simulink subsystem "Global_2_Local_Path"  (R2022b)
settings: Solver=VariableStepAuto  StartTime=0.0  StopTime=10.0  RelTol=1e-3
settings Model: Creator=User  LastModifiedBy=User

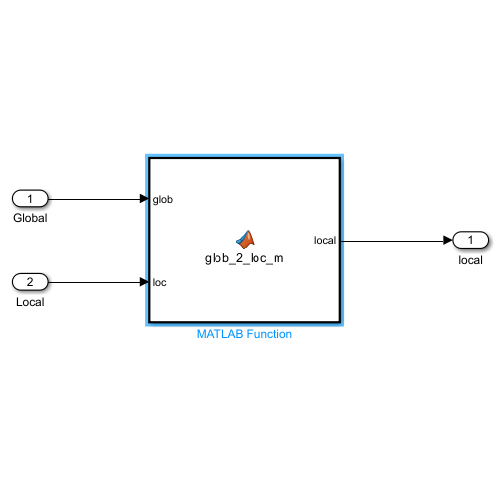
[thumbnail: Simulink's stored preview of the top-level diagram]
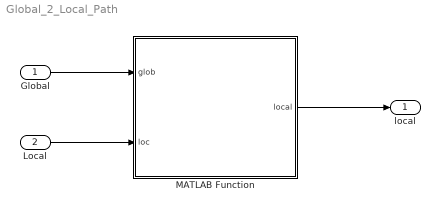
== system Global_2_Local_Path ==
  Global : Inport
  Local : Inport  Port=2
  MATLAB Function : MATLAB Function  TreatAsAtomicUnit=on
  local : Outport
  wires:
  Global/1 -> MATLAB Function/1(glob)
  Local/1 -> MATLAB Function/2(loc)
  MATLAB Function/1(local) -> local/1

== matlab function Global_2_Local_Path/MATLAB Function ==
  data: glob input; local output; loc input
function local = glob_2_loc_m(glob,loc)
    local = glob_2_loc(glob,loc);
    
end
